simulink model "Ex2_model"  (R2024b)
settings: Solver=VariableStepAuto  StartTime=0.0  StopTime=50  RelTol=1e-3
values from neighbouring files (symbols this model uses):
  A = [0, 1; 0, -10]    [Ex1_script.m]    (also in Ex3_script.m = [0, 1; -2, -40]; Ex4_script.m = [0,1; 0,-20])
  B = [0; 120]    [Ex1_script.m]    (also in Ex3_script.m = [0; 40]; Ex4_script.m = [0; 60])
  C = [1, 0]    [Ex1_script.m]    (also in Ex3_script.m; Ex4_script.m)
  D = 0    [Ex1_script.m]    (also in Ex3_script.m; Ex4_script.m)
  Gamma = Bo*Ts    [Ex2_script.m]
  H = Co    [Ex2_script.m]
  J = Do    [Ex2_script.m]
  K = Kr    [Ex2_script.m]    (also in Ex3_script.m = Ke(2:3); Ex4_script.m = Ke(4:5))
  Ki = Kp/Ti    [Ex1_script.m]    (also in Ex2_script.m = Ke(1); Ex3_script.m = Ke(1))
  nominal_robust = 1    [Ex2_script.m]
  Nu = ff(3)    [Ex2_script.m]    (also in Ex3_script.m)
  Nx = ff(1:2)    [Ex2_script.m]    (also in Ex3_script.m)
  Phi = eye(2)+Ao*Ts    [Ex2_script.m]
  Ts = tr/250    (= 0.001)    [Ex2_script.m]    (also in Ex3_script.m = 1e-05)
undefined symbols (not defined in the file or in its folder): DiscIntNeverNeededParam
settings Model: Creator=pries  LastModifiedBy=pries

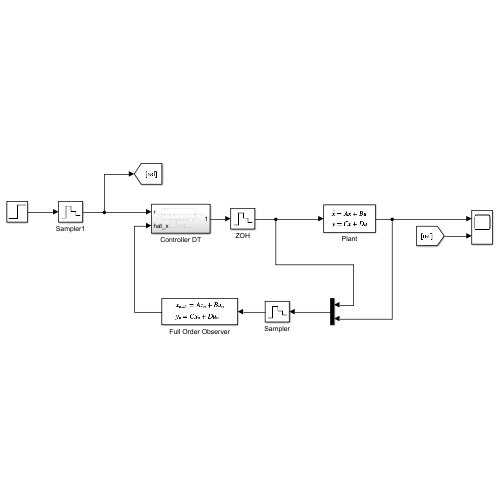
[thumbnail: Simulink's stored preview of the top-level diagram]
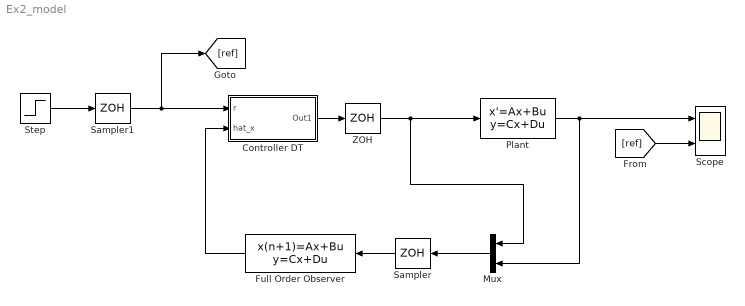
== system Ex2_model ==
  Controller DT : Subsystem
  Full Order Observer : DiscreteStateSpace  A=Phi  B=Gamma  C=H  D=J  SampleTime=Ts
  Mux : Mux  Inputs=2
  Plant : StateSpace  A=A  B=B  C=C  D=D  InitialCondition=0
  Sampler : ZeroOrderHold  SampleTime=Ts
  Sampler1 : ZeroOrderHold  SampleTime=Ts
  Scope : Scope  NumInputPorts=2
  Step : Step  Time=0  SampleTime=0
  ZOH : ZeroOrderHold  SampleTime=Ts
  wires:
  Mux/1 -> Sampler/1
  Controller DT/1(Out1) -> ZOH/1
  Plant/1 -> Mux/2, Scope/1
  Step/1 -> Sampler1/1
  Full Order Observer/1 -> Controller DT/2(hat_x)
  [ref] -> Scope/2
  Sampler/1 -> Full Order Observer/1
  Sampler1/1 -> [ref], Controller DT/1(r)
  ZOH/1 -> Plant/1, Mux/1

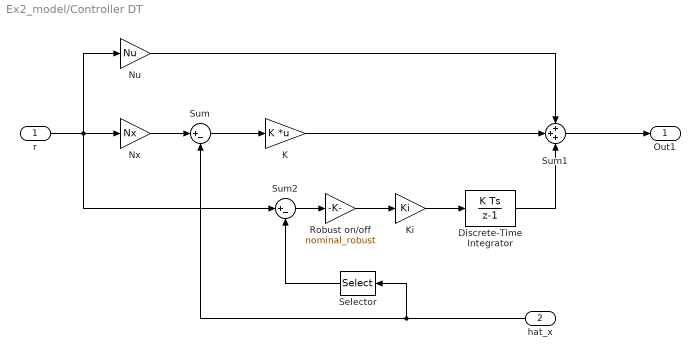
== system Ex2_model/Controller DT ==
  r : Inport
  hat_x : Inport  Port=2
  Discrete-Time Integrator : DiscreteIntegrator  SampleTime=Ts  ICPrevOutput=DiscIntNeverNeededParam  ICPrevScaledInput=DiscIntNeverNeededParam
  K : Gain  Gain=K  Multiplication=Matrix(K*u)
  Ki : Gain  Gain=Ki
  Nu : Gain  Gain=Nu
  Nx : Gain  Gain=Nx
  Robust on/off : Gain  Gain=nominal_robust
  Selector : Selector  InputPortWidth=2  IndexOptions=Index vector (dialog)  Indices=1  OutputSizes=1
  Sum : Sum  Inputs=|+-
  Sum1 : Sum  Inputs=+++
  Sum2 : Sum  Inputs=|+-
  Out1 : Outport
  wires:
  r/1 -> Sum2/1, Nu/1, Nx/1
  Nx/1 -> Sum/1
  Sum/1 -> K/1
  K/1 -> Sum1/2
  Nu/1 -> Sum1/1
  hat_x/1 -> Selector/1, Sum/2
  Sum1/1 -> Out1/1
  Ki/1 -> Discrete-Time Integrator/1
  Robust on/off/1 -> Ki/1
  Discrete-Time Integrator/1 -> Sum1/3
  Sum2/1 -> Robust on/off/1
  Selector/1 -> Sum2/2
